simulink model "RP_Obstacle_Environment_Gamepad"  (R2018a)
settings: Solver=ode23t  StartTime=0.0  StopTime=inf  FixedStep=0.01  RelTol=1e-3  EnableMultiTasking=on
InitFcn:
  | RPInit
model workspace (MAT data in the model file):
  mapForSim.obsMap = [0 0 0 0 0 0 0 0 0 0 0 0 ... (2621440 elements, 2048x1280)]
  mapForSim.scaleFactor = 256
  mapForSim.simMap = robotics.BinaryOccupancyGrid
  mapForSim.simMap.Grid = [1 1 1 1 1 1 1 1 1 1 1 1 ... (2621440 elements, 2048x1280)]
  mapForSim.simMap.GridSize = [2048 1280]
  mapForSim.simMap.Resolution = 256
  occGrid = robotics.BinaryOccupancyGrid
  occGrid.Grid = [1 1 1 1 1 1 1 1 1 1 1 1 ... (2621440 elements, 2048x1280)]
  occGrid.GridSize = [2048 1280]
  occGrid.Resolution = 256
libraries: RoboticsPlayground x9, vexarmcortexlib x2
settings Model: EnablePacing=on  ExtModeTrigDuration=25  Creator=scastro  LastModifiedBy=josea
settings SolverCC: AlgebraicLoopSolver=LineSearch
settings DataIOCC: LimitDataPoints=on
settings OptimizationCC: PassReuseOutputArgsAs=Individual arguments  MaxStackSize=64
settings DebuggingCC: ParameterTunabilityLossMsg=error  AllowSymbolicDim=off  SFUnexpectedBacktrackingDiag=warning  SFNoUnconditionalDefaultTransitionDiag=warning  SFExecutionAtInitializationDiag=none
settings HardwareCC: ProdBitPerPointer=32  ProdBitPerSizeT=32  ProdBitPerPtrDiffT=32  ProdLargestAtomicInteger=Long  ProdLargestAtomicFloat=Double  ProdWordSize=32  ProdHWDeviceType=ARM Compatible->ARM Cortex
settings SFSimCC: MATLABDynamicMemAlloc=off
settings RTWCC: SystemTargetFile=ert.tlc  HardwareBoard=ARM Cortex-based VEX Microcontroller  TLCOptions="-aInlineSetEventsForThisBaseRateFcn=TLC_FALSE -aSuppressMultiTaskScheduler=TLC_FALSE  -aRateBasedStepFcn=0"  TemplateMakefile=ert_default_tmf  GenerateReport=on  Toolchain=GNU Tools for VEX ARM Cortex  IncludeHyperlinkInReport=on  LaunchReport=on  GenerateTraceInfo=on  GenerateTraceReport=on  GenerateTraceReportSl=on  GenerateTraceReportSf=on  GenerateTraceReportEml=on
settings CodeAppCC: ForceParamTrailComments=on  IgnoreCustomStorageClasses=off  OperatorAnnotations=on  SimulinkDataObjDesc=on  SFDataObjDesc=on  InsertBlockDesc=on
settings ConfigComp: CovMetricSettings=dw  CovHtmlReporting=on  CovSaveCumulativeToWorkspaceVar=on  CovSaveSingleToWorkspaceVar=on  CovExternalEMLEnable=off  CovSFcnEnable=off
settings SimscapeCC: SimscapeNominalValues="[{\"value\":\"10\",\"unit\":\"V\"},{\"value\":\"1\",\"unit\":\"A\"},{\"value\":\"10\",\"unit\":\"N*m\"},{\"value\":\"10\",\"unit\":\"bar\"},{\"value\":\"100\",\"unit\":\"kJ/kg\"},{\"value\":\"1\",\"unit\":\"kW\"},{\"value\":\"300\",\"unit\":\"K\"},{\"value\":\"100\",\"unit\":\"cm^3/s\"},{\"value\":\"1\",\"unit\":\"kN\"},{\"value\":\"1\",\"unit\":\"g/cm^3\"},{\"value\":\"1\",\"unit\":\"l\"},{\"value\":\"1\",\"unit\":\"cm^2\"},{\"value\":\"60\",\"unit\":\"Hz\"}]"  SimscapeLogDataHistory=10000
settings ConfigurationSet: Description=SimMechanics 2G
settings DiagnosticsConfigSet: SimMechanicsRigidlyBoundBlock=none
settings ExplorerConfigSet: InternalSimMechanicsExplorerSettings="<ExplorerConfiguration><canonicalview>default</canonicalview><AnimationSetting><BasePlaybackSpeed>1.0</BasePlaybackSpeed><PlaybackSpeedFactor>1.0</PlaybackSpeedFactor></AnimationSetting><TilePanel><TileInfo><Tiles Columns=\"2\" Count=\"3\" Rows=\"2\"><Column Weight=\"0.5\"/><Column Weight=\"0.5\"/><Row Weight=\"0.5558\"/><Row Weight=\"0.4442\"/><Tile Height=\"1\" Width=\"2\" X=\"0\" Y=\"0\"/><Tile Height=\"1\" Width=\"1\" X=\"0\" Y=\"1\"/><Tile Height=\"1\" Width=\"1\" X=\"1\" Y=\"1\"/></Tiles></TileInfo><SceneInfo><SceneViewer><BGColor><R>0.60000002384185791</R><G>0.60000002384185791</G><B>0.60000002384185791</B></BGColor><Camera><DoPerspective>off</DoPerspective><Position><X>3.77812343469301437</X><Y>-3.77812335288872925</Y><Z>3.7781233369241094</Z></Position><Center><X>-2.07139932301910341e-08</X><Y>1.02518278512960765e-07</Y><Z>-1.18482898008922e-07</Z></Center><Up><X>-0.408248290463863073</X><Y>0.408248290463863073</Y><Z>0.816496580927726145</Z></Up><ViewLimDist>1</ViewLimDist><YLim>2.86778095960617074</YLim><XLim>6.75102172519388599</XLim></Camera></SceneViewer><SceneViewer><BGColor><R>0.60000002384185791</R><G>0.60000002384185791</G><B>0.60000002384185791</B></BGColor><Camera><DoPerspective>on</DoPerspective><Position><X>0.025687663764123736</X><Y>0.399310018201750161</Y><Z>0.453907703599162216</Z></Position><Center><X>0.541332794341274459</X><Y>-0.386267680610761999</Y><Z>0.111887560273493503</Z></Center><Up><X>0.187679478974392022</X><Y>-0.285926899071094254</Y><Z>0.939692620785908428</Z></Up><ViewLimDist>1</ViewLimDist><YLim>0.466307658154998583</YLim><XLim>0.683848507606772515</XLim></Camera></SceneViewer><SceneViewer><BGColor><R>0.60000002384185791</R><G>0.60000002384185791</G><B>0.60000002384185791</B></BGColor><Camera><DoPerspective>off</DoPerspective><Position><X>-0.018234885227883621</X><Y>-0.0300165861003731764</Y><Z>37.6782594368875863</Z></Position><Center><X>-0.018234885227883621</X><Y>-0.0300165861003731764</Y><Z>0.069999846435872648</Z></Center><Up><X>0</X><Y>1</Y><Z>-0</Z></Up><ViewLimDist>1</ViewLimDist><YLim>5.44437616630040022</YLim><XLim>7.98427486888250648</XLim></Camera></SceneViewer></SceneInfo></TilePanel><MechEditorPanel><Cameras><Camera><Id>Camera1</Id><Value><Name>RobotView</Name><NativeCamera><PositionTrackingFeature>Obstacle_Environment.Robot.Body.RobotCamera.F</PositionTrackingFeature><CenterTrackingFeature>Obstacle_Environment.Robot.Body.RobotCamera.F</CenterTrackingFeature><UpVectorTrackingFeature>Obstacle_Environment.Robot.Body.RobotCamera.F</UpVectorTrackingFeature><CenterTrackingOrigin>off</CenterTrackingOrigin><CenterTrackingDirection>+X</CenterTrackingDirection><UpVectorTrackingDirection>+Z</UpVectorTrackingDirection></NativeCamera></Value></Camera></Cameras><GfxPanelCameraMap><MapElement CameraMLId=\"Camera1\" GfxPanelIndex=\"1\"/></GfxPanelCameraMap><VideoCreator><PlaybackSpeedRatio>1.0</PlaybackSpeedRatio><FrameRate>30</FrameRate><VideoFormat>Motion JPEG AVI</VideoFormat><FrameSize>auto</FrameSize></VideoCreator></MechEditorPanel></ExplorerConfiguration>"

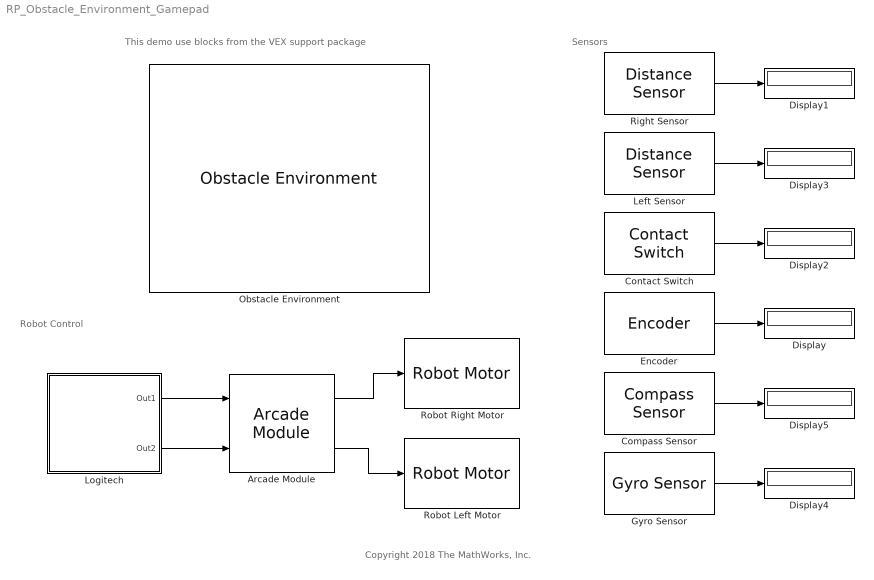
== system RP_Obstacle_Environment_Gamepad ==
  note: Robot Control
  note: Sensors
  note: Copyright 2018 The MathWorks, Inc.
  note: This demo use blocks from the VEX support package
  Arcade Module : vexarmcortexlib/Utilities/Arcade Module
      settings: SourceProductName=Simulink Coder Support Package for ARM Cortex-based VEX Microcontroller  SourceProductBaseCode=EC_VEX_MICRO
  Compass Sensor : RoboticsPlayground/Basic Sensors and Actuators/Compass Sensor  robotId=1  sensorTs=0.1
      settings: SourceProductName=Robotics Playground
  Contact Switch : RoboticsPlayground/Basic Sensors and Actuators/Contact Switch  robotId=1  trigDist=0.02  sensOff=[0.25 0]  sensOffDeg=0  sensorTs=0.1
      settings: SourceProductName=Robotics Playground
  Display{,1..5} (6 alike) : Display
  Encoder : RoboticsPlayground/Basic Sensors and Actuators/Encoder  robotId=1  motorChoice=1  rstChoice=No reset  ticks=180  detectDir=off  sensorTs=0.1
      settings: SourceProductName=Robotics Playground
  Gyro Sensor : RoboticsPlayground/Basic Sensors and Actuators/Gyro Sensor  robotId=1  sensor=Body Center  sensorTs=0.1
      settings: SourceProductName=Robotics Playground
  Left Sensor : RoboticsPlayground/Basic Sensors and Actuators/Distance Sensor  robotId=1  maxSenRange=2  minSenRange=0.02  senRes=0.01  sensOff=[0.18 0.18]  sensOffDeg=45  sensorTs=0.1
      settings: SourceProductName=Robotics Playground
  Logitech : Subsystem
      mask Display:
      | pic = imread('Gamepad_Controller.png');
      | image(pic);
  Obstacle Environment : RoboticsPlayground/Environments/Obstacle Environment  obs1=on  obsPose1="[0.14251      3.2953]"  obsWidth1=4.0293  obsLength1=0.31625  obs2=on  obsPose2="[1.8233    -0.44119]"  obsWidth2=0.24597  obsLength2=5.7042  obs3=on  obsPose3="[-0.33772     -3.1938]"  obsWidth3=3.3734  obsLength3=0.55051  obs4=on  obsPose4="[-0.43729    -0.97413]"  obsWidth4=3.1274  obsLength4=0.37482  obs5=off  obsPose5="[1.6535    -0.67545]"  obsWidth5=0.39824  obsLength5=0.71449  obs6=off  obsPose6="[3.1293     -1.6301]"  obsWidth6=0.60322  obsLength6=0.47438  obs7=off  obsPose7=[2 2]  obsWidth7=0.8  obsLength7=0.4  obs8=off  obsPose8=[2 2]  obsWidth8=0.8  obsLength8=0.4  obs9=off  obsPose9=[2 2]  obsWidth9=0.8  obsLength9=0.4  obs10=off  obsPose10=[2 2]  obsWidth10=0.8  obsLength10=0.4  arenaLength=5  arenaWidth=8  robotId=1  wheelBase=0.5  wheelRadius=0.1  robotColor=[0 0 0.5]  startPose=[-1.4 0]
      settings: SourceProductName=Robotics Playground
  Right Sensor : RoboticsPlayground/Basic Sensors and Actuators/Distance Sensor  robotId=1  maxSenRange=2  minSenRange=0.02  senRes=0.01  sensOff=[0.18 -0.18]  sensOffDeg=-45  sensorTs=0.1
      settings: SourceProductName=Robotics Playground
  Robot Left Motor : RoboticsPlayground/Basic Sensors and Actuators/Robot Motor  OverrideUsingVariant=Rbt1R  robotId=1  motorChoice=1
      settings: SourceProductName=Robotics Playground
  Robot Right Motor : RoboticsPlayground/Basic Sensors and Actuators/Robot Motor  OverrideUsingVariant=Rbt1R  robotId=1  motorChoice=2
      settings: SourceProductName=Robotics Playground
  wires:
  Arcade Module/1 -> Robot Right Motor/1
  Arcade Module/2 -> Robot Left Motor/1
  Logitech/1(Out1) -> Arcade Module/1
  Logitech/2(Out2) -> Arcade Module/2
  Encoder/1 -> Display/1
  Right Sensor/1 -> Display1/1
  Contact Switch/1 -> Display2/1
  Left Sensor/1 -> Display3/1
  Gyro Sensor/1 -> Display4/1
  Compass Sensor/1 -> Display5/1

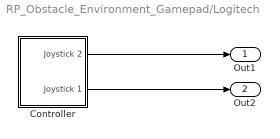
== system RP_Obstacle_Environment_Gamepad/Logitech ==
  Controller : Subsystem
  Out1 : Outport
  Out2 : Outport  Port=2
  wires:
  Controller/1(Joystick 2) -> Out1/1
  Controller/2(Joystick 1) -> Out2/1

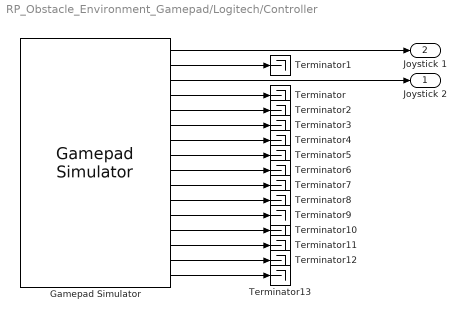
== system RP_Obstacle_Environment_Gamepad/Logitech/Controller ==
  Gamepad Simulator : vexarmcortexlib/Utilities/Gamepad Simulator  WhichPad=Logitech Gamepad  JoyId=1
      settings: SourceProductName=Simulink Coder Support Package for ARM Cortex-based VEX Microcontroller  SourceProductBaseCode=EC_VEX_MICRO
  Terminator{,1..13} (14 alike) : Terminator
  Joystick 2 : Outport
  Joystick 1 : Outport  Port=2
  wires:
  Gamepad Simulator/1 -> Joystick 1/1
  Gamepad Simulator/3 -> Joystick 2/1
  Gamepad Simulator/4 -> Terminator/1
  Gamepad Simulator/2 -> Terminator1/1
  Gamepad Simulator/5 -> Terminator2/1
  Gamepad Simulator/6 -> Terminator3/1
  Gamepad Simulator/7 -> Terminator4/1
  Gamepad Simulator/8 -> Terminator5/1
  Gamepad Simulator/9 -> Terminator6/1
  Gamepad Simulator/10 -> Terminator7/1
  Gamepad Simulator/11 -> Terminator8/1
  Gamepad Simulator/12 -> Terminator9/1
  Gamepad Simulator/13 -> Terminator10/1
  Gamepad Simulator/14 -> Terminator11/1
  Gamepad Simulator/15 -> Terminator12/1
  Gamepad Simulator/16 -> Terminator13/1
